simulink model "ctrl_typeB"  (R2016b)
settings: Solver=ode45  StartTime=0.0  StopTime=10.0  RelTol=1e-3  EnableMultiTasking=on
undefined symbols (not defined in the file): gain_act_GASBF, gain_act_GASF0, gain_act_GASF1, gain_act_LIM, gain_act_LIP, gain_act_LTM, gain_act_PIM, gain_act_PTM, gain_act_RIM, gain_act_TIM, gain_act_TIP, gain_act_VIM, gain_act_YIM, gain_act_YIP, gain_act_YTM, gain_GASBF, gain_GASF0, gain_GASF1, gain_global_LIM, gain_global_LIP, gain_global_LTM, gain_LIM, gain_LIP, gain_LTM, gain_oplev_PIM, gain_oplev_YIM, gain_PIM, gain_PTM, gain_RIM, gain_TIM, gain_TIP, gain_VIM, gain_YIM, gain_YIP, gain_YTM, sys1
libraries: cstblocks x26, simulink x3
settings Model: Creator=TAMA Project  LastModifiedBy=miyo
settings DataIOCC: LimitDataPoints=on  SaveFormat=Array  SignalLoggingSaveFormat=ModelDataLogs
settings OptimizationCC: ExpressionDepthLimit=2147483647  LifeSpan=inf
settings DebuggingCC: UnderspecifiedInitializationDetection=Classic  MergeDetectMultiDrivingBlocksExec=none  FcnCallInpInsideContextMsg=warning  StateNameClashWarn=warning  SFUnexpectedBacktrackingDiag=warning  SFNoUnconditionalDefaultTransitionDiag=warning  SFExecutionAtInitializationDiag=none
settings HardwareCC: ProdBitPerPointer=32  ProdBitPerSizeT=32  ProdBitPerPtrDiffT=32  ProdLargestAtomicFloat=None  ProdIntDivRoundTo=Undefined  ProdEndianess=Unspecified  ProdWordSize=32  ProdHWDeviceType=32-bit Generic
settings ModelReferenceCC: PropagateSignalLabelsOutOfModel=off
settings GRTTargetCC: TargetLangStandard=C89/C90 (ANSI)  GeneratePreprocessorConditionals=Disable all  CombineOutputUpdateFcns=off  GRTInterface=on
settings ConfigComp: CovMetricSettings=dw  CovHtmlReporting=on  CovSaveCumulativeToWorkspaceVar=on  CovSaveSingleToWorkspaceVar=on  CovExternalEMLEnable=off  CovSFcnEnable=off

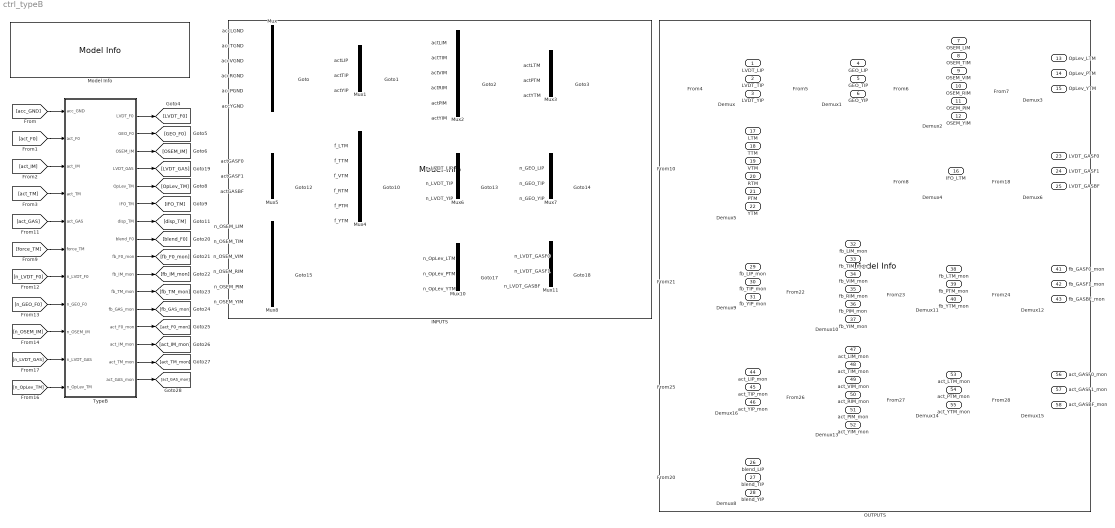
== system ctrl_typeB ==
  accLGND : Inport
  accTGND : Inport  Port=2
  accVGND : Inport  Port=3
  accRGND : Inport  Port=4
  accPGND : Inport  Port=5
  accYGND : Inport  Port=6
  actLIP : Inport  Port=7
  actTIP : Inport  Port=8
  actYIP : Inport  Port=9
  actLIM : Inport  Port=10
  actTIM : Inport  Port=11
  actVIM : Inport  Port=12
  actRIM : Inport  Port=13
  actPIM : Inport  Port=14
  actYIM : Inport  Port=15
  actLTM : Inport  Port=16
  actPTM : Inport  Port=17
  actYTM : Inport  Port=18
  f_LTM : Inport  Port=19
  f_TTM : Inport  Port=20
  f_VTM : Inport  Port=21
  f_RTM : Inport  Port=22
  f_PTM : Inport  Port=23
  f_YTM : Inport  Port=24
  actGASF0 : Inport  Port=25
  actGASF1 : Inport  Port=26
  actGASBF : Inport  Port=27
  n_LVDT_LIP : Inport  Port=28
  n_LVDT_TIP : Inport  Port=29
  n_LVDT_YIP : Inport  Port=30
  n_GEO_LIP : Inport  Port=31
  n_GEO_TIP : Inport  Port=32
  n_GEO_YIP : Inport  Port=33
  n_OSEM_LIM : Inport  Port=34
  n_OSEM_TIM : Inport  Port=35
  n_OSEM_VIM : Inport  Port=36
  n_OSEM_RIM : Inport  Port=37
  n_OSEM_PIM : Inport  Port=38
  n_OSEM_YIM : Inport  Port=39
  n_OpLev_LTM : Inport  Port=40
  n_OpLev_PTM : Inport  Port=41
  n_OpLev_YTM : Inport  Port=42
  n_LVDT_GASF0 : Inport  Port=43
  n_LVDT_GASF1 : Inport  Port=44
  n_LVDT_GASBF : Inport  Port=45
  Demux{,1,3,6,8..9,11..12,14..16} (11 alike) : Demux  Outputs=3
  Demux{2,5,10,13} (4 alike) : Demux  Outputs=6
  Demux4 : Demux  Outputs=1
  INPUTS : simulink/Model-Wide Utilities/Model Info  Frame=on  DisplayStringWithTags=Model Info  HorizontalTextAlignment=Left  LeftAlignmentValue=0.02  SourceBlockDiagram=ctrl_typeB  TagMaxNumber=20
  Model Info : simulink/Model-Wide Utilities/Model Info  Frame=on  DisplayStringWithTags=|  HorizontalTextAlignment=Left  LeftAlignmentValue=0.02  SourceBlockDiagram=ctrl_typeB  TagMaxNumber=20
      | [MODEL INFORMATION]
      | 
      | ModelName: %<ModelName>
      | LastUpdate : %<LastModificationDate>
      | 
      | TypeB1 prototype control model
  Mux{,2,4,8} (4 alike) : Mux  Inputs=6
  Mux{1,3,5..7,10..11} (7 alike) : Mux  Inputs=3
  OUTPUTS : simulink/Model-Wide Utilities/Model Info  Frame=on  DisplayStringWithTags=Model Info  HorizontalTextAlignment=Left  LeftAlignmentValue=0.02  SourceBlockDiagram=ctrl_typeB  TagMaxNumber=20
  TypeB : Subsystem
  LVDT_LIP : Outport
  LVDT_TIP : Outport  Port=2
  LVDT_YIP : Outport  Port=3
  GEO_LIP : Outport  Port=4
  GEO_TIP : Outport  Port=5
  GEO_YIP : Outport  Port=6
  OSEM_LIM : Outport  Port=7
  OSEM_TIM : Outport  Port=8
  OSEM_VIM : Outport  Port=9
  OSEM_RIM : Outport  Port=10
  OSEM_PIM : Outport  Port=11
  OSEM_YIM : Outport  Port=12
  OpLev_LTM : Outport  Port=13
  OpLev_PTM : Outport  Port=14
  OpLev_YTM : Outport  Port=15
  IFO_LTM : Outport  Port=16
  LTM : Outport  Port=17
  TTM : Outport  Port=18
  VTM : Outport  Port=19
  RTM : Outport  Port=20
  PTM : Outport  Port=21
  YTM : Outport  Port=22
  LVDT_GASF0 : Outport  Port=23
  LVDT_GASF1 : Outport  Port=24
  LVDT_GASBF : Outport  Port=25
  blend_LIP : Outport  Port=26
  blend_TIP : Outport  Port=27
  blend_YIP : Outport  Port=28
  fb_LIP_mon : Outport  Port=29
  fb_TIP_mon : Outport  Port=30
  fb_YIP_mon : Outport  Port=31
  fb_LIM_mon : Outport  Port=32
  fb_TIM_mon : Outport  Port=33
  fb_VIM_mon : Outport  Port=34
  fb_RIM_mon : Outport  Port=35
  fb_PIM_mon : Outport  Port=36
  fb_YIM_mon : Outport  Port=37
  fb_LTM_mon : Outport  Port=38
  fb_PTM_mon : Outport  Port=39
  fb_YTM_mon : Outport  Port=40
  fb_GASF0_mon : Outport  Port=41
  fb_GASF1_mon : Outport  Port=42
  fb_GASBF_mon : Outport  Port=43
  act_LIP_mon : Outport  Port=44
  act_TIP_mon : Outport  Port=45
  act_YIP_mon : Outport  Port=46
  act_LIM_mon : Outport  Port=47
  act_TIM_mon : Outport  Port=48
  act_VIM_mon : Outport  Port=49
  act_RIM_mon : Outport  Port=50
  act_PIM_mon : Outport  Port=51
  act_YIM_mon : Outport  Port=52
  act_LTM_mon : Outport  Port=53
  act_PTM_mon : Outport  Port=54
  act_YTM_mon : Outport  Port=55
  act_GASF0_mon : Outport  Port=56
  act_GASF1_mon : Outport  Port=57
  act_GASBF_mon : Outport  Port=58
  wires:
  accLGND/1 -> Mux/1
  accTGND/1 -> Mux/2
  accVGND/1 -> Mux/3
  accRGND/1 -> Mux/4
  accPGND/1 -> Mux/5
  accYGND/1 -> Mux/6
  Mux/1 -> [acc_GND]
  actLIP/1 -> Mux1/1
  actTIP/1 -> Mux1/2
  actYIP/1 -> Mux1/3
  Mux1/1 -> [act_F0]
  actLIM/1 -> Mux2/1
  actTIM/1 -> Mux2/2
  actVIM/1 -> Mux2/3
  actRIM/1 -> Mux2/4
  actPIM/1 -> Mux2/5
  actYIM/1 -> Mux2/6
  Mux2/1 -> [act_IM]
  actLTM/1 -> Mux3/1
  actPTM/1 -> Mux3/2
  actYTM/1 -> Mux3/3
  Mux3/1 -> [act_TM]
  [acc_GND] -> TypeB/1(acc_GND)
  [act_F0] -> TypeB/2(act_F0)
  [act_IM] -> TypeB/3(act_IM)
  [act_TM] -> TypeB/4(act_TM)
  TypeB/1(LVDT_F0) -> [LVDT_F0]
  TypeB/2(GEO_F0) -> [GEO_F0]
  TypeB/3(OSEM_IM) -> [OSEM_IM]
  TypeB/5(OpLev_TM) -> [OpLev_TM]
  [LVDT_F0] -> Demux/1
  Demux/1 -> LVDT_LIP/1
  Demux/2 -> LVDT_TIP/1
  Demux/3 -> LVDT_YIP/1
  [GEO_F0] -> Demux1/1
  Demux1/1 -> GEO_LIP/1
  Demux1/2 -> GEO_TIP/1
  Demux1/3 -> GEO_YIP/1
  [OSEM_IM] -> Demux2/1
  Demux2/1 -> OSEM_LIM/1
  Demux2/2 -> OSEM_TIM/1
  Demux2/3 -> OSEM_VIM/1
  Demux2/4 -> OSEM_RIM/1
  Demux2/5 -> OSEM_PIM/1
  Demux2/6 -> OSEM_YIM/1
  [OpLev_TM] -> Demux3/1
  TypeB/6(IFO_TM) -> [IFO_TM]
  [IFO_TM] -> Demux4/1
  Demux4/1 -> IFO_LTM/1
  f_LTM/1 -> Mux4/1
  f_TTM/1 -> Mux4/2
  f_VTM/1 -> Mux4/3
  Mux4/1 -> [force_TM]
  f_YTM/1 -> Mux4/6
  f_PTM/1 -> Mux4/5
  f_RTM/1 -> Mux4/4
  [force_TM] -> TypeB/6(force_TM)
  TypeB/7(disp_TM) -> [disp_TM]
  [disp_TM] -> Demux5/1
  Demux5/1 -> LTM/1
  Demux5/2 -> TTM/1
  Demux5/3 -> VTM/1
  Demux5/4 -> RTM/1
  Demux5/5 -> PTM/1
  Demux5/6 -> YTM/1
  actGASF0/1 -> Mux5/1
  actGASF1/1 -> Mux5/2
  actGASBF/1 -> Mux5/3
  Mux5/1 -> [act_GAS]
  [act_GAS] -> TypeB/5(act_GAS)
  n_LVDT_LIP/1 -> Mux6/1
  n_LVDT_TIP/1 -> Mux6/2
  n_LVDT_YIP/1 -> Mux6/3
  Mux6/1 -> [n_LVDT_F0]
  n_GEO_LIP/1 -> Mux7/1
  n_GEO_TIP/1 -> Mux7/2
  n_GEO_YIP/1 -> Mux7/3
  Mux7/1 -> [n_GEO_F0]
  n_OSEM_LIM/1 -> Mux8/1
  n_OSEM_TIM/1 -> Mux8/2
  n_OSEM_VIM/1 -> Mux8/3
  n_OSEM_RIM/1 -> Mux8/4
  n_OSEM_PIM/1 -> Mux8/5
  n_OSEM_YIM/1 -> Mux8/6
  Mux8/1 -> [n_OSEM_IM]
  Mux10/1 -> [n_OpLev_TM]
  [n_LVDT_F0] -> TypeB/7(n_LVDT_F0)
  [n_GEO_F0] -> TypeB/8(n_GEO_F0)
  [n_OSEM_IM] -> TypeB/9(n_OSEM_IM)
  n_LVDT_GASF0/1 -> Mux11/1
  n_LVDT_GASF1/1 -> Mux11/2
  n_LVDT_GASBF/1 -> Mux11/3
  Mux11/1 -> [n_LVDT_GAS]
  [n_LVDT_GAS] -> TypeB/10(n_LVDT_GAS)
  TypeB/4(LVDT_GAS) -> [LVDT_GAS]
  [LVDT_GAS] -> Demux6/1
  Demux6/1 -> LVDT_GASF0/1
  Demux6/2 -> LVDT_GASF1/1
  Demux6/3 -> LVDT_GASBF/1
  [n_OpLev_TM] -> TypeB/11(n_OpLev_TM)
  TypeB/8(blend_F0) -> [blend_F0]
  TypeB/9(fb_F0_mon) -> [fb_F0_mon]
  TypeB/10(fb_IM_mon) -> [fb_IM_mon]
  TypeB/11(fb_TM_mon) -> [fb_TM_mon]
  TypeB/12(fb_GAS_mon) -> [fb_GAS_mon]
  TypeB/13(act_F0_mon) -> [act_F0_mon]
  TypeB/14(act_IM_mon) -> [act_IM_mon]
  TypeB/15(act_TM_mon) -> [act_TM_mon]
  TypeB/16(act_GAS_mon) -> [act_GAS_mon]
  [blend_F0] -> Demux8/1
  Demux8/1 -> blend_LIP/1
  Demux8/2 -> blend_TIP/1
  Demux8/3 -> blend_YIP/1
  [fb_F0_mon] -> Demux9/1
  Demux9/1 -> fb_LIP_mon/1
  Demux9/2 -> fb_TIP_mon/1
  Demux9/3 -> fb_YIP_mon/1
  [fb_IM_mon] -> Demux10/1
  Demux10/1 -> fb_LIM_mon/1
  Demux10/2 -> fb_TIM_mon/1
  Demux10/3 -> fb_VIM_mon/1
  Demux10/4 -> fb_RIM_mon/1
  Demux10/5 -> fb_PIM_mon/1
  Demux10/6 -> fb_YIM_mon/1
  [fb_TM_mon] -> Demux11/1
  Demux11/1 -> fb_LTM_mon/1
  Demux11/2 -> fb_PTM_mon/1
  Demux11/3 -> fb_YTM_mon/1
  [fb_GAS_mon] -> Demux12/1
  Demux12/1 -> fb_GASF0_mon/1
  Demux12/2 -> fb_GASF1_mon/1
  Demux12/3 -> fb_GASBF_mon/1
  [act_F0_mon] -> Demux16/1
  Demux16/1 -> act_LIP_mon/1
  Demux16/2 -> act_TIP_mon/1
  Demux16/3 -> act_YIP_mon/1
  [act_IM_mon] -> Demux13/1
  Demux13/1 -> act_LIM_mon/1
  Demux13/2 -> act_TIM_mon/1
  Demux13/3 -> act_VIM_mon/1
  Demux13/4 -> act_RIM_mon/1
  Demux13/5 -> act_PIM_mon/1
  Demux13/6 -> act_YIM_mon/1
  [act_TM_mon] -> Demux14/1
  Demux14/1 -> act_LTM_mon/1
  Demux14/2 -> act_PTM_mon/1
  Demux14/3 -> act_YTM_mon/1
  [act_GAS_mon] -> Demux15/1
  Demux15/1 -> act_GASF0_mon/1
  Demux15/2 -> act_GASF1_mon/1
  Demux15/3 -> act_GASBF_mon/1
  n_OpLev_LTM/1 -> Mux10/1
  n_OpLev_PTM/1 -> Mux10/2
  n_OpLev_YTM/1 -> Mux10/3
  Demux3/1 -> OpLev_LTM/1
  Demux3/2 -> OpLev_PTM/1
  Demux3/3 -> OpLev_YTM/1

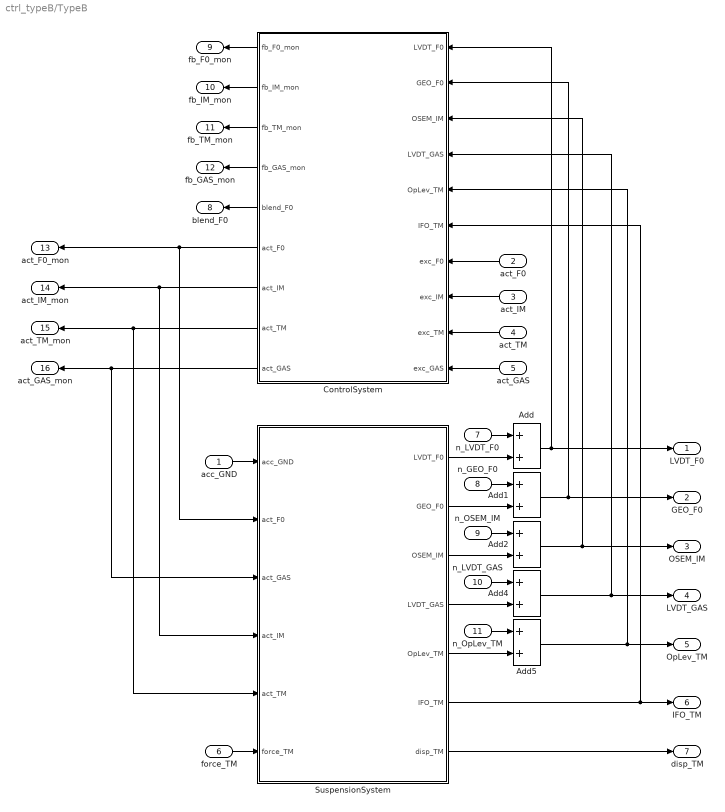
== system ctrl_typeB/TypeB ==
  acc_GND : Inport
  act_F0 : Inport  Port=2
  act_IM : Inport  Port=3
  act_TM : Inport  Port=4
  act_GAS : Inport  Port=5
  force_TM : Inport  Port=6
  n_LVDT_F0 : Inport  Port=7
  n_GEO_F0 : Inport  Port=8
  n_OSEM_IM : Inport  Port=9
  n_LVDT_GAS : Inport  Port=10
  n_OpLev_TM : Inport  Port=11
  Add{,1..2,4..5} (5 alike) : Sum
  ControlSystem : Subsystem
  SuspensionSystem : Subsystem
  LVDT_F0 : Outport
  GEO_F0 : Outport  Port=2
  OSEM_IM : Outport  Port=3
  LVDT_GAS : Outport  Port=4
  OpLev_TM : Outport  Port=5
  IFO_TM : Outport  Port=6
  disp_TM : Outport  Port=7
  blend_F0 : Outport  Port=8
  fb_F0_mon : Outport  Port=9
  fb_IM_mon : Outport  Port=10
  fb_TM_mon : Outport  Port=11
  fb_GAS_mon : Outport  Port=12
  act_F0_mon : Outport  Port=13
  act_IM_mon : Outport  Port=14
  act_TM_mon : Outport  Port=15
  act_GAS_mon : Outport  Port=16
  wires:
  acc_GND/1 -> SuspensionSystem/1(acc_GND)
  force_TM/1 -> SuspensionSystem/6(force_TM)
  SuspensionSystem/7(disp_TM) -> disp_TM/1
  SuspensionSystem/1(LVDT_F0) -> Add/2
  SuspensionSystem/2(GEO_F0) -> Add1/2
  n_GEO_F0/1 -> Add1/1
  n_LVDT_F0/1 -> Add/1
  SuspensionSystem/3(OSEM_IM) -> Add2/2
  n_OSEM_IM/1 -> Add2/1
  SuspensionSystem/6(IFO_TM) -> IFO_TM/1, ControlSystem/6(IFO_TM)
  Add/1 -> LVDT_F0/1, ControlSystem/1(LVDT_F0)
  Add1/1 -> ControlSystem/2(GEO_F0), GEO_F0/1
  Add2/1 -> ControlSystem/3(OSEM_IM), OSEM_IM/1
  n_LVDT_GAS/1 -> Add4/1
  SuspensionSystem/4(LVDT_GAS) -> Add4/2
  n_OpLev_TM/1 -> Add5/1
  SuspensionSystem/5(OpLev_TM) -> Add5/2
  Add4/1 -> ControlSystem/4(LVDT_GAS), LVDT_GAS/1
  Add5/1 -> ControlSystem/5(OpLev_TM), OpLev_TM/1
  ControlSystem/5(blend_F0) -> blend_F0/1
  act_GAS/1 -> ControlSystem/10(exc_GAS)
  act_TM/1 -> ControlSystem/9(exc_TM)
  act_IM/1 -> ControlSystem/8(exc_IM)
  act_F0/1 -> ControlSystem/7(exc_F0)
  ControlSystem/6(act_F0) -> act_F0_mon/1, SuspensionSystem/2(act_F0)
  ControlSystem/7(act_IM) -> SuspensionSystem/4(act_IM), act_IM_mon/1
  ControlSystem/8(act_TM) -> act_TM_mon/1, SuspensionSystem/5(act_TM)
  ControlSystem/9(act_GAS) -> SuspensionSystem/3(act_GAS), act_GAS_mon/1
  ControlSystem/1(fb_F0_mon) -> fb_F0_mon/1
  ControlSystem/2(fb_IM_mon) -> fb_IM_mon/1
  ControlSystem/3(fb_TM_mon) -> fb_TM_mon/1
  ControlSystem/4(fb_GAS_mon) -> fb_GAS_mon/1

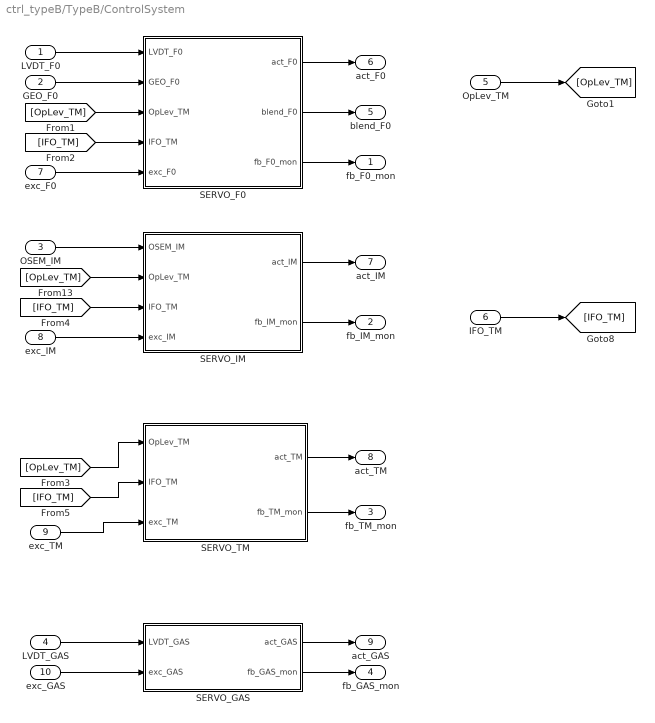
== system ctrl_typeB/TypeB/ControlSystem ==
  LVDT_F0 : Inport
  GEO_F0 : Inport  Port=2
  OSEM_IM : Inport  Port=3
  LVDT_GAS : Inport  Port=4
  OpLev_TM : Inport  Port=5
  IFO_TM : Inport  Port=6
  exc_F0 : Inport  Port=7
  exc_IM : Inport  Port=8
  exc_TM : Inport  Port=9
  exc_GAS : Inport  Port=10
  SERVO_F0 : Subsystem
  SERVO_GAS : Subsystem
  SERVO_IM : Subsystem
  SERVO_TM : Subsystem
  fb_F0_mon : Outport
  fb_IM_mon : Outport  Port=2
  fb_TM_mon : Outport  Port=3
  fb_GAS_mon : Outport  Port=4
  blend_F0 : Outport  Port=5
  act_F0 : Outport  Port=6
  act_IM : Outport  Port=7
  act_TM : Outport  Port=8
  act_GAS : Outport  Port=9
  wires:
  IFO_TM/1 -> [IFO_TM]
  LVDT_F0/1 -> SERVO_F0/1(LVDT_F0)
  GEO_F0/1 -> SERVO_F0/2(GEO_F0)
  SERVO_F0/1(act_F0) -> act_F0/1
  SERVO_IM/1(act_IM) -> act_IM/1
  OSEM_IM/1 -> SERVO_IM/1(OSEM_IM)
  LVDT_GAS/1 -> SERVO_GAS/1(LVDT_GAS)
  SERVO_GAS/1(act_GAS) -> act_GAS/1
  SERVO_TM/1(act_TM) -> act_TM/1
  OpLev_TM/1 -> [OpLev_TM]
  [OpLev_TM] -> SERVO_IM/2(OpLev_TM)
  [IFO_TM] -> SERVO_F0/4(IFO_TM)
  [IFO_TM] -> SERVO_IM/3(IFO_TM)
  [OpLev_TM] -> SERVO_F0/3(OpLev_TM)
  SERVO_F0/2(blend_F0) -> blend_F0/1
  exc_F0/1 -> SERVO_F0/5(exc_F0)
  exc_IM/1 -> SERVO_IM/4(exc_IM)
  exc_GAS/1 -> SERVO_GAS/2(exc_GAS)
  SERVO_F0/3(fb_F0_mon) -> fb_F0_mon/1
  SERVO_IM/2(fb_IM_mon) -> fb_IM_mon/1
  SERVO_TM/2(fb_TM_mon) -> fb_TM_mon/1
  SERVO_GAS/2(fb_GAS_mon) -> fb_GAS_mon/1
  [OpLev_TM] -> SERVO_TM/1(OpLev_TM)
  [IFO_TM] -> SERVO_TM/2(IFO_TM)
  exc_TM/1 -> SERVO_TM/3(exc_TM)

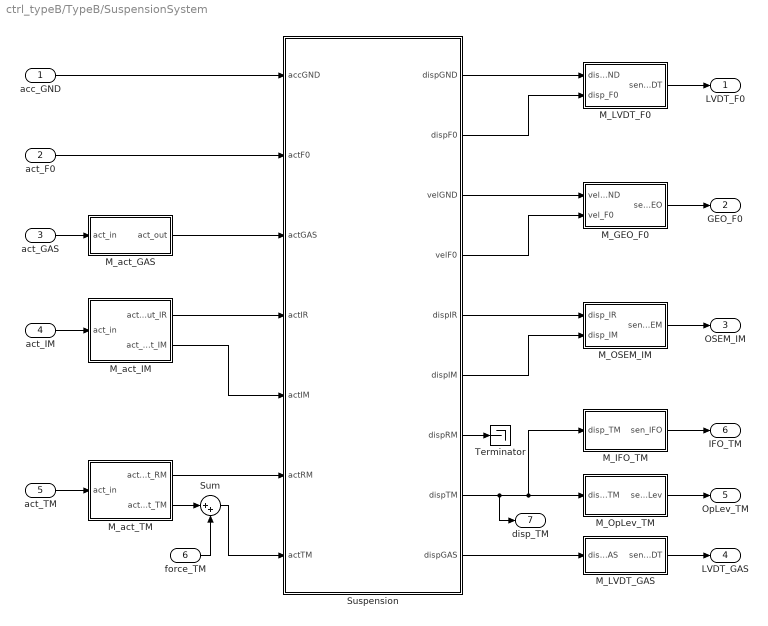
== system ctrl_typeB/TypeB/SuspensionSystem ==
  acc_GND : Inport
  act_F0 : Inport  Port=2
  act_GAS : Inport  Port=3
  act_IM : Inport  Port=4
  act_TM : Inport  Port=5
  force_TM : Inport  Port=6
  M_GEO_F0 : Subsystem
  M_IFO_TM : Subsystem
  M_LVDT_F0 : Subsystem
  M_LVDT_GAS : Subsystem
  M_OSEM_IM : Subsystem
  M_OpLev_TM : Subsystem
  M_act_GAS : Subsystem
  M_act_IM : Subsystem
  M_act_TM : Subsystem
  Sum : Sum  Inputs=|++
  Suspension : Subsystem
  Terminator : Terminator
  LVDT_F0 : Outport
  GEO_F0 : Outport  Port=2
  OSEM_IM : Outport  Port=3
  LVDT_GAS : Outport  Port=4
  OpLev_TM : Outport  Port=5
  IFO_TM : Outport  Port=6
  disp_TM : Outport  Port=7
  wires:
  acc_GND/1 -> Suspension/1(accGND)
  act_F0/1 -> Suspension/2(actF0)
  act_IM/1 -> M_act_IM/1(act_in)
  M_act_IM/1(act_out_IR) -> Suspension/4(actIR)
  M_act_IM/2(act_out_IM) -> Suspension/5(actIM)
  act_TM/1 -> M_act_TM/1(act_in)
  Sum/1 -> Suspension/7(actTM)
  M_act_TM/2(act_out_TM) -> Sum/1
  force_TM/1 -> Sum/2
  M_act_GAS/1(act_out) -> Suspension/3(actGAS)
  act_GAS/1 -> M_act_GAS/1(act_in)
  Suspension/1(dispGND) -> M_LVDT_F0/1(disp_GND)
  Suspension/2(dispF0) -> M_LVDT_F0/2(disp_F0)
  M_LVDT_F0/1(sen_LVDT) -> LVDT_F0/1
  Suspension/3(velGND) -> M_GEO_F0/1(vel_GND)
  Suspension/4(velF0) -> M_GEO_F0/2(vel_F0)
  M_GEO_F0/1(sen_GEO) -> GEO_F0/1
  Suspension/5(dispIR) -> M_OSEM_IM/1(disp_IR)
  Suspension/6(dispIM) -> M_OSEM_IM/2(disp_IM)
  M_OSEM_IM/1(sen_OSEM) -> OSEM_IM/1
  Suspension/8(dispTM) -> disp_TM/1, M_IFO_TM/1(disp_TM), M_OpLev_TM/1(disp_TM)
  Suspension/9(dispGAS) -> M_LVDT_GAS/1(disp_GAS)
  M_LVDT_GAS/1(sen_LVDT) -> LVDT_GAS/1
  M_IFO_TM/1(sen_IFO) -> IFO_TM/1
  M_OpLev_TM/1(sen_OpLev) -> OpLev_TM/1
  Suspension/7(dispRM) -> Terminator/1
  M_act_TM/1(act_out_RM) -> Suspension/6(actRM)

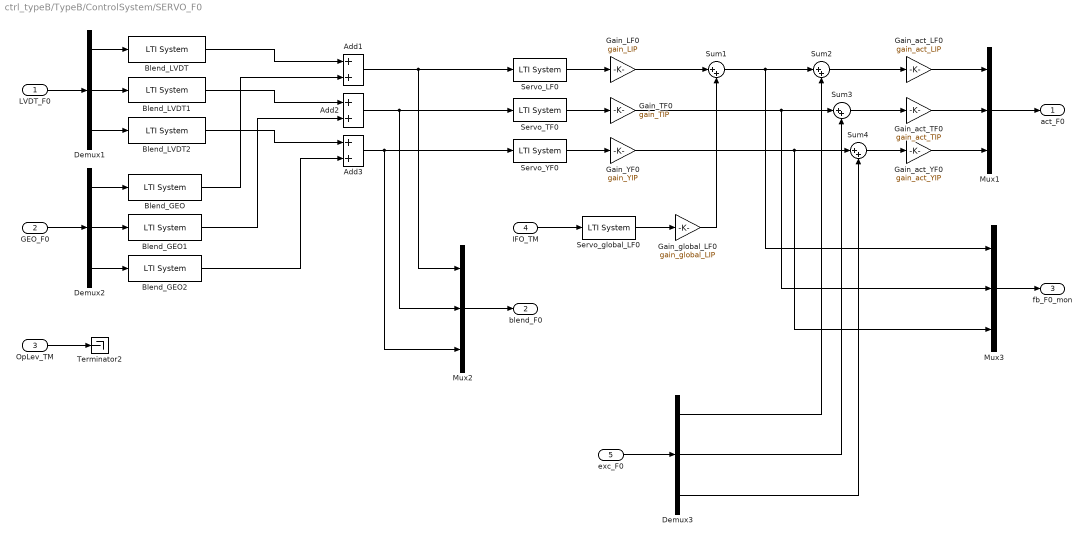
== system ctrl_typeB/TypeB/ControlSystem/SERVO_F0 ==
  LVDT_F0 : Inport
  GEO_F0 : Inport  Port=2
  OpLev_TM : Inport  Port=3
  IFO_TM : Inport  Port=4
  exc_F0 : Inport  Port=5
  Add1 : Sum
  Add2 : Sum
  Add3 : Sum
  Blend_GEO : cstblocks/LTI System  sys=blend_GEO  IC=[]
  Blend_GEO1 : cstblocks/LTI System  sys=blend_GEO  IC=[]
  Blend_GEO2 : cstblocks/LTI System  sys=blend_GEO  IC=[]
  Blend_LVDT : cstblocks/LTI System  sys=blend_LVDT  IC=[]
  Blend_LVDT1 : cstblocks/LTI System  sys=blend_LVDT  IC=[]
  Blend_LVDT2 : cstblocks/LTI System  sys=blend_LVDT  IC=[]
  Demux1 : Demux  Outputs=3
  Demux2 : Demux  Outputs=3
  Demux3 : Demux  Outputs=3
  Gain_LF0 : Gain  Gain=gain_LIP
  Gain_TF0 : Gain  Gain=gain_TIP
  Gain_YF0 : Gain  Gain=gain_YIP
  Gain_act_LF0 : Gain  Gain=gain_act_LIP
  Gain_act_TF0 : Gain  Gain=gain_act_TIP
  Gain_act_YF0 : Gain  Gain=gain_act_YIP
  Gain_global_LF0 : Gain  Gain=gain_global_LIP
  Mux1 : Mux  Inputs=3
  Mux2 : Mux  Inputs=3
  Mux3 : Mux  Inputs=3
  Servo_LF0 : cstblocks/LTI System  sys=servo_LIP  IC=[]
  Servo_TF0 : cstblocks/LTI System  sys=servo_TIP  IC=[]
  Servo_YF0 : cstblocks/LTI System  sys=servo_YIP  IC=[]
  Servo_global_LF0 : cstblocks/LTI System  sys=servo_global_LIP  IC=[]
  Sum{1..4} (4 alike) : Sum  Inputs=|++
  Terminator2 : Terminator
  act_F0 : Outport
  blend_F0 : Outport  Port=2
  fb_F0_mon : Outport  Port=3
  wires:
  Blend_LVDT/1 -> Add1/1
  IFO_TM/1 -> Servo_global_LF0/1
  Mux1/1 -> act_F0/1
  LVDT_F0/1 -> Demux1/1
  GEO_F0/1 -> Demux2/1
  Demux1/1 -> Blend_LVDT/1
  Demux1/2 -> Blend_LVDT1/1
  Demux1/3 -> Blend_LVDT2/1
  Demux2/1 -> Blend_GEO/1
  Demux2/2 -> Blend_GEO1/1
  Demux2/3 -> Blend_GEO2/1
  Blend_LVDT1/1 -> Add2/1
  Blend_LVDT2/1 -> Add3/1
  Blend_GEO/1 -> Add1/2
  Blend_GEO1/1 -> Add2/2
  Blend_GEO2/1 -> Add3/2
  Add1/1 -> Servo_LF0/1, Mux2/1
  Add2/1 -> Servo_TF0/1, Mux2/2
  Add3/1 -> Servo_YF0/1, Mux2/3
  OpLev_TM/1 -> Terminator2/1
  Servo_LF0/1 -> Gain_LF0/1
  Gain_LF0/1 -> Sum1/1
  Servo_TF0/1 -> Gain_TF0/1
  Servo_YF0/1 -> Gain_YF0/1
  Servo_global_LF0/1 -> Gain_global_LF0/1
  Gain_global_LF0/1 -> Sum1/2
  Gain_act_LF0/1 -> Mux1/1
  Gain_act_TF0/1 -> Mux1/2
  Gain_act_YF0/1 -> Mux1/3
  Mux2/1 -> blend_F0/1
  Gain_TF0/1 -> Mux3/2, Sum3/1
  Sum2/1 -> Gain_act_LF0/1
  Sum1/1 -> Mux3/1, Sum2/1
  Sum3/1 -> Gain_act_TF0/1
  exc_F0/1 -> Demux3/1
  Demux3/1 -> Sum2/2
  Demux3/2 -> Sum3/2
  Demux3/3 -> Sum4/2
  Gain_YF0/1 -> Mux3/3, Sum4/1
  Sum4/1 -> Gain_act_YF0/1
  Mux3/1 -> fb_F0_mon/1

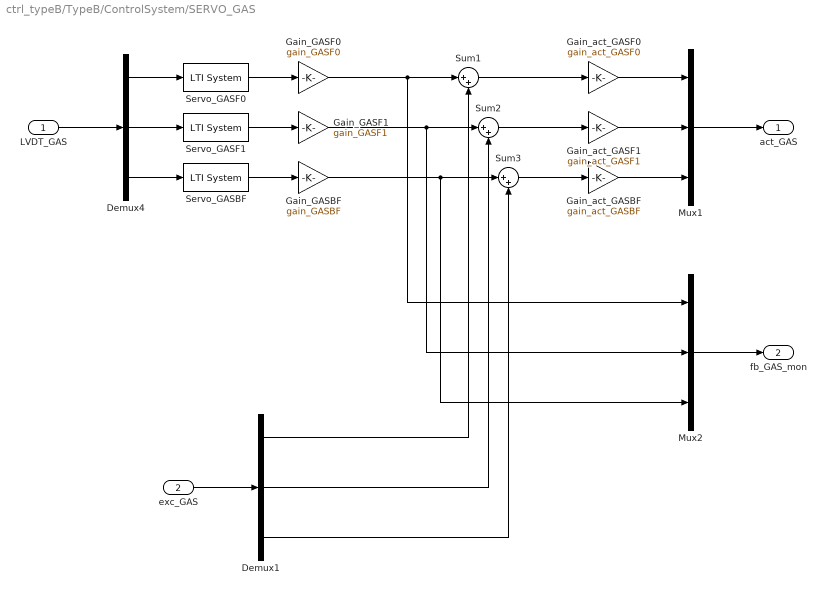
== system ctrl_typeB/TypeB/ControlSystem/SERVO_GAS ==
  LVDT_GAS : Inport
  exc_GAS : Inport  Port=2
  Demux1 : Demux  Outputs=3
  Demux4 : Demux  Outputs=3
  Gain_GASBF : Gain  Gain=gain_GASBF
  Gain_GASF0 : Gain  Gain=gain_GASF0
  Gain_GASF1 : Gain  Gain=gain_GASF1
  Gain_act_GASBF : Gain  Gain=gain_act_GASBF
  Gain_act_GASF0 : Gain  Gain=gain_act_GASF0
  Gain_act_GASF1 : Gain  Gain=gain_act_GASF1
  Mux1 : Mux  Inputs=3
  Mux2 : Mux  Inputs=3
  Servo_GASBF : cstblocks/LTI System  sys=servo_GASBF  IC=[]
  Servo_GASF0 : cstblocks/LTI System  sys=servo_GASF0  IC=[]
  Servo_GASF1 : cstblocks/LTI System  sys=servo_GASF1  IC=[]
  Sum1 : Sum  Inputs=|++
  Sum2 : Sum  Inputs=|++
  Sum3 : Sum  Inputs=|++
  act_GAS : Outport
  fb_GAS_mon : Outport  Port=2
  wires:
  Demux4/1 -> Servo_GASF0/1
  Demux4/2 -> Servo_GASF1/1
  Demux4/3 -> Servo_GASBF/1
  Servo_GASF0/1 -> Gain_GASF0/1
  Servo_GASF1/1 -> Gain_GASF1/1
  Servo_GASBF/1 -> Gain_GASBF/1
  Gain_act_GASF0/1 -> Mux1/1
  Gain_act_GASF1/1 -> Mux1/2
  Gain_act_GASBF/1 -> Mux1/3
  LVDT_GAS/1 -> Demux4/1
  Mux1/1 -> act_GAS/1
  exc_GAS/1 -> Demux1/1
  Gain_GASF0/1 -> Mux2/1, Sum1/1
  Sum1/1 -> Gain_act_GASF0/1
  Gain_GASF1/1 -> Mux2/2, Sum2/1
  Sum2/1 -> Gain_act_GASF1/1
  Gain_GASBF/1 -> Mux2/3, Sum3/1
  Sum3/1 -> Gain_act_GASBF/1
  Demux1/1 -> Sum1/2
  Demux1/2 -> Sum2/2
  Demux1/3 -> Sum3/2
  Mux2/1 -> fb_GAS_mon/1

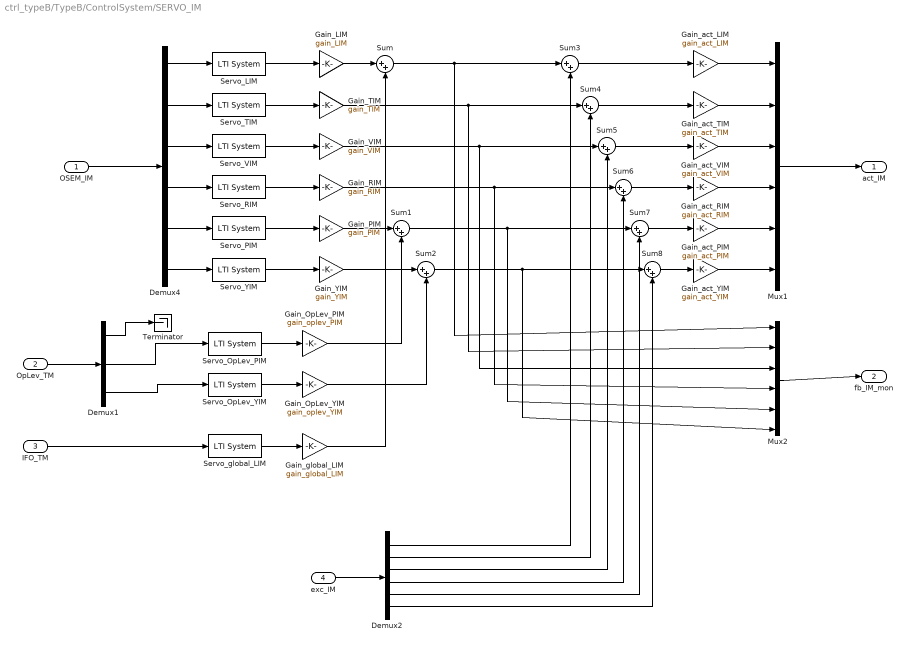
== system ctrl_typeB/TypeB/ControlSystem/SERVO_IM ==
  OSEM_IM : Inport
  OpLev_TM : Inport  Port=2
  IFO_TM : Inport  Port=3
  exc_IM : Inport  Port=4
  Demux1 : Demux  Outputs=3
  Demux2 : Demux  Outputs=6
  Demux4 : Demux  Outputs=6
  Gain_LIM : Gain  Gain=gain_LIM
  Gain_OpLev_PIM : Gain  Gain=gain_oplev_PIM
  Gain_OpLev_YIM : Gain  Gain=gain_oplev_YIM
  Gain_PIM : Gain  Gain=gain_PIM
  Gain_RIM : Gain  Gain=gain_RIM
  Gain_TIM : Gain  Gain=gain_TIM
  Gain_VIM : Gain  Gain=gain_VIM
  Gain_YIM : Gain  Gain=gain_YIM
  Gain_act_LIM : Gain  Gain=gain_act_LIM
  Gain_act_PIM : Gain  Gain=gain_act_PIM
  Gain_act_RIM : Gain  Gain=gain_act_RIM
  Gain_act_TIM : Gain  Gain=gain_act_TIM
  Gain_act_VIM : Gain  Gain=gain_act_VIM
  Gain_act_YIM : Gain  Gain=gain_act_YIM
  Gain_global_LIM : Gain  Gain=gain_global_LIM
  Mux1 : Mux  Inputs=6
  Mux2 : Mux  Inputs=6
  Servo_LIM : cstblocks/LTI System  sys=servo_LIM  IC=[]
  Servo_OpLev_PIM : cstblocks/LTI System  sys=servo_oplev_PIM  IC=[]
  Servo_OpLev_YIM : cstblocks/LTI System  sys=servo_oplev_YIM  IC=[]
  Servo_PIM : cstblocks/LTI System  sys=servo_PIM  IC=[]
  Servo_RIM : cstblocks/LTI System  sys=servo_RIM  IC=[]
  Servo_TIM : cstblocks/LTI System  sys=servo_TIM  IC=[]
  Servo_VIM : cstblocks/LTI System  sys=servo_VIM  IC=[]
  Servo_YIM : cstblocks/LTI System  sys=servo_YIM  IC=[]
  Servo_global_LIM : cstblocks/LTI System  sys=servo_global_LIM  IC=[]
  Sum{,1..8} (9 alike) : Sum  Inputs=|++
  Terminator : Terminator
  act_IM : Outport
  fb_IM_mon : Outport  Port=2
  wires:
  Demux4/1 -> Servo_LIM/1
  Demux4/2 -> Servo_TIM/1
  Demux4/3 -> Servo_VIM/1
  Servo_LIM/1 -> Gain_LIM/1
  Servo_TIM/1 -> Gain_TIM/1
  Servo_VIM/1 -> Gain_VIM/1
  Mux1/1 -> act_IM/1
  Gain_act_LIM/1 -> Mux1/1
  Gain_act_TIM/1 -> Mux1/2
  Gain_act_VIM/1 -> Mux1/3
  OSEM_IM/1 -> Demux4/1
  Servo_RIM/1 -> Gain_RIM/1
  Servo_PIM/1 -> Gain_PIM/1
  Servo_YIM/1 -> Gain_YIM/1
  Demux4/4 -> Servo_RIM/1
  Demux4/5 -> Servo_PIM/1
  Demux4/6 -> Servo_YIM/1
  Gain_act_RIM/1 -> Mux1/4
  Gain_act_PIM/1 -> Mux1/5
  Gain_act_YIM/1 -> Mux1/6
  OpLev_TM/1 -> Demux1/1
  IFO_TM/1 -> Servo_global_LIM/1
  Gain_LIM/1 -> Sum/1
  Servo_global_LIM/1 -> Gain_global_LIM/1
  Gain_PIM/1 -> Sum1/1
  Gain_YIM/1 -> Sum2/1
  Gain_global_LIM/1 -> Sum/2
  Servo_OpLev_PIM/1 -> Gain_OpLev_PIM/1
  Servo_OpLev_YIM/1 -> Gain_OpLev_YIM/1
  Gain_OpLev_PIM/1 -> Sum1/2
  Gain_OpLev_YIM/1 -> Sum2/2
  Sum/1 -> Sum3/1, Mux2/1
  Sum3/1 -> Gain_act_LIM/1
  Gain_TIM/1 -> Mux2/2, Sum4/1
  Sum4/1 -> Gain_act_TIM/1
  Gain_VIM/1 -> Mux2/3, Sum5/1
  Sum5/1 -> Gain_act_VIM/1
  Gain_RIM/1 -> Sum6/1, Mux2/4
  Sum6/1 -> Gain_act_RIM/1
  Sum1/1 -> Sum7/1, Mux2/5
  Sum7/1 -> Gain_act_PIM/1
  Sum2/1 -> Sum8/1, Mux2/6
  Sum8/1 -> Gain_act_YIM/1
  Demux2/1 -> Sum3/2
  Demux2/2 -> Sum4/2
  Demux2/3 -> Sum5/2
  Demux2/4 -> Sum6/2
  Demux2/5 -> Sum7/2
  Demux2/6 -> Sum8/2
  exc_IM/1 -> Demux2/1
  Mux2/1 -> fb_IM_mon/1
  Demux1/3 -> Servo_OpLev_YIM/1
  Demux1/2 -> Servo_OpLev_PIM/1
  Demux1/1 -> Terminator/1

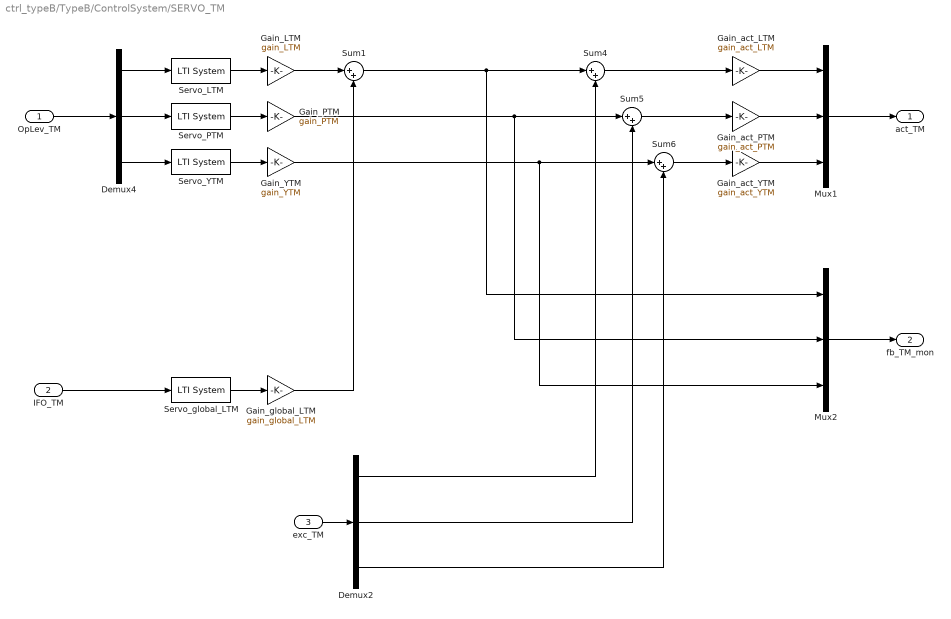
== system ctrl_typeB/TypeB/ControlSystem/SERVO_TM ==
  OpLev_TM : Inport
  IFO_TM : Inport  Port=2
  exc_TM : Inport  Port=3
  Demux2 : Demux  Outputs=3
  Demux4 : Demux  Outputs=3
  Gain_LTM : Gain  Gain=gain_LTM
  Gain_PTM : Gain  Gain=gain_PTM
  Gain_YTM : Gain  Gain=gain_YTM
  Gain_act_LTM : Gain  Gain=gain_act_LTM
  Gain_act_PTM : Gain  Gain=gain_act_PTM
  Gain_act_YTM : Gain  Gain=gain_act_YTM
  Gain_global_LTM : Gain  Gain=gain_global_LTM
  Mux1 : Mux  Inputs=3
  Mux2 : Mux  Inputs=3
  Servo_LTM : cstblocks/LTI System  sys=servo_LTM  IC=[]
  Servo_PTM : cstblocks/LTI System  sys=servo_PTM  IC=[]
  Servo_YTM : cstblocks/LTI System  sys=servo_YTM  IC=[]
  Servo_global_LTM : cstblocks/LTI System  sys=servo_global_LTM  IC=[]
  Sum{1,4..6} (4 alike) : Sum  Inputs=|++
  act_TM : Outport
  fb_TM_mon : Outport  Port=2
  wires:
  Demux4/1 -> Servo_LTM/1
  Demux4/2 -> Servo_PTM/1
  Demux4/3 -> Servo_YTM/1
  Servo_LTM/1 -> Gain_LTM/1
  Servo_PTM/1 -> Gain_PTM/1
  Servo_YTM/1 -> Gain_YTM/1
  OpLev_TM/1 -> Demux4/1
  Mux1/1 -> act_TM/1
  IFO_TM/1 -> Servo_global_LTM/1
  Servo_global_LTM/1 -> Gain_global_LTM/1
  Gain_LTM/1 -> Sum1/1
  Gain_global_LTM/1 -> Sum1/2
  Gain_act_LTM/1 -> Mux1/1
  Gain_act_PTM/1 -> Mux1/2
  Gain_act_YTM/1 -> Mux1/3
  Sum1/1 -> Mux2/1, Sum4/1
  Sum4/1 -> Gain_act_LTM/1
  Gain_PTM/1 -> Mux2/2, Sum5/1
  Sum5/1 -> Gain_act_PTM/1
  Gain_YTM/1 -> Mux2/3, Sum6/1
  Sum6/1 -> Gain_act_YTM/1
  exc_TM/1 -> Demux2/1
  Demux2/1 -> Sum4/2
  Demux2/2 -> Sum5/2
  Demux2/3 -> Sum6/2
  Mux2/1 -> fb_TM_mon/1

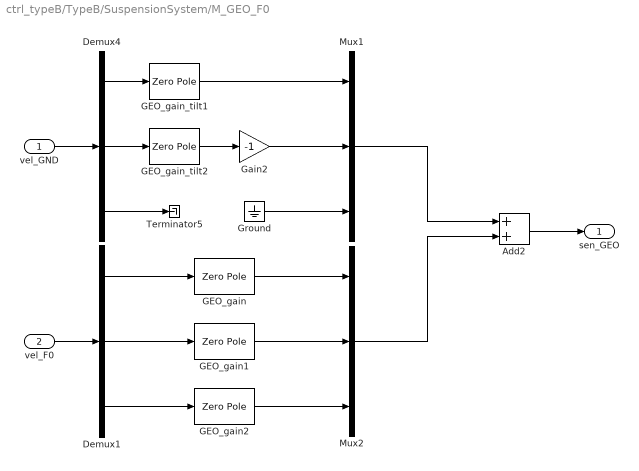
== system ctrl_typeB/TypeB/SuspensionSystem/M_GEO_F0 ==
  vel_GND : Inport
  vel_F0 : Inport  Port=2
  Add2 : Sum
  Demux1 : Demux  Outputs=3
  Demux4 : Demux  Outputs=3
  GEO_gain : ZeroPole  Zeros=[0 0]  Poles=[-2.13+1i*5.19 -2.13-1i*5.19]
  GEO_gain1 : ZeroPole  Zeros=[0 0]  Poles=[-2.13+1i*5.19 -2.13-1i*5.19]
  GEO_gain2 : ZeroPole  Zeros=[0 0]  Poles=[-2.13+1i*5.19 -2.13-1i*5.19]
  GEO_gain_tilt1 : ZeroPole  Zeros=[]  Poles=[-2.13+1i*5.19 -2.13-1i*5.19]
  GEO_gain_tilt2 : ZeroPole  Zeros=[]  Poles=[-2.13+1i*5.19 -2.13-1i*5.19]
  Gain2 : Gain  Gain=-1
  Ground : Ground
  Mux1 : Mux  Inputs=3
  Mux2 : Mux  Inputs=3
  Terminator5 : Terminator
  sen_GEO : Outport
  wires:
  Add2/1 -> sen_GEO/1
  Mux1/1 -> Add2/1
  Demux4/2 -> GEO_gain_tilt2/1
  Demux4/1 -> GEO_gain_tilt1/1
  Gain2/1 -> Mux1/2
  Ground/1 -> Mux1/3
  GEO_gain_tilt1/1 -> Mux1/1
  vel_GND/1 -> Demux4/1
  GEO_gain_tilt2/1 -> Gain2/1
  vel_F0/1 -> Demux1/1
  Demux1/1 -> GEO_gain/1
  Demux1/2 -> GEO_gain1/1
  Demux1/3 -> GEO_gain2/1
  GEO_gain/1 -> Mux2/1
  GEO_gain1/1 -> Mux2/2
  GEO_gain2/1 -> Mux2/3
  Mux2/1 -> Add2/2
  Demux4/3 -> Terminator5/1

== system ctrl_typeB/TypeB/SuspensionSystem/M_IFO_TM ==
  disp_TM : Inport
  Add2 : Sum  Inputs=++++
  Demux4 : Demux  Outputs=6
  Gain1 : Gain  Gain=1/300
  Gain2 : Gain  Gain=1e-3
  Gain3 : Gain  Gain=1e-3
  Terminator1 : Terminator
  Terminator3 : Terminator
  sen_IFO : Outport
  wires:
  disp_TM/1 -> Demux4/1
  Demux4/4 -> Terminator3/1
  Demux4/3 -> Gain1/1
  Demux4/2 -> Terminator1/1
  Add2/1 -> sen_IFO/1
  Demux4/1 -> Add2/1
  Gain1/1 -> Add2/2
  Demux4/5 -> Gain2/1
  Gain3/1 -> Add2/4
  Gain2/1 -> Add2/3
  Demux4/6 -> Gain3/1

== system ctrl_typeB/TypeB/SuspensionSystem/M_LVDT_F0 ==
  disp_GND : Inport
  disp_F0 : Inport  Port=2
  Add2 : Sum  Inputs=-+
  sen_LVDT : Outport
  wires:
  Add2/1 -> sen_LVDT/1
  disp_F0/1 -> Add2/2
  disp_GND/1 -> Add2/1

== system ctrl_typeB/TypeB/SuspensionSystem/M_LVDT_GAS ==
  disp_GAS : Inport
  Add1 : Sum  Inputs=-+
  Add2 : Sum  Inputs=-+
  Add3 : Sum  Inputs=-+
  Demux4 : Demux
  Mux3 : Mux  Inputs=3
  sen_LVDT : Outport
  wires:
  disp_GAS/1 -> Demux4/1
  Demux4/1 -> Add2/1
  Demux4/2 -> Add2/2, Add1/1
  Demux4/3 -> Add3/1, Add1/2
  Demux4/4 -> Add3/2
  Add2/1 -> Mux3/1
  Add1/1 -> Mux3/2
  Add3/1 -> Mux3/3
  Mux3/1 -> sen_LVDT/1

== system ctrl_typeB/TypeB/SuspensionSystem/M_OSEM_IM ==
  disp_IR : Inport
  disp_IM : Inport  Port=2
  Add1 : Sum
  Add2 : Sum  Inputs=+-
  Add3 : Sum  Inputs=-+
  Demux4 : Demux  Outputs=6
  Gain : Gain  Gain=76e-3
  Gain1 : Gain  Gain=76e-3
  Mux3 : Mux  Inputs=6
  sen_OSEM : Outport
  wires:
  disp_IM/1 -> Add3/2
  disp_IR/1 -> Demux4/1
  Demux4/6 -> Mux3/6
  Mux3/1 -> Add3/1
  Add3/1 -> sen_OSEM/1
  Demux4/1 -> Add2/1
  Demux4/2 -> Add1/1
  Demux4/3 -> Mux3/3
  Demux4/4 -> Gain/1, Mux3/4
  Demux4/5 -> Gain1/1, Mux3/5
  Gain1/1 -> Add2/2
  Gain/1 -> Add1/2
  Add1/1 -> Mux3/2
  Add2/1 -> Mux3/1

== system ctrl_typeB/TypeB/SuspensionSystem/M_OpLev_TM ==
  disp_TM : Inport
  Demux4 : Demux  Outputs=6
  Mux3 : Mux  Inputs=3
  Terminator1 : Terminator
  Terminator2 : Terminator
  Terminator3 : Terminator
  sen_OpLev : Outport
  wires:
  disp_TM/1 -> Demux4/1
  Mux3/1 -> sen_OpLev/1
  Demux4/4 -> Terminator3/1
  Demux4/3 -> Terminator2/1
  Demux4/2 -> Terminator1/1
  Demux4/1 -> Mux3/1
  Demux4/5 -> Mux3/2
  Demux4/6 -> Mux3/3

== system ctrl_typeB/TypeB/SuspensionSystem/M_act_GAS ==
  act_in : Inport
  Add1 : Sum  Inputs=+-
  Add2 : Sum  Inputs=+-
  Demux4 : Demux  Outputs=3
  Mux3 : Mux  Inputs=3
  act_out : Outport
  wires:
  act_in/1 -> Demux4/1
  Mux3/1 -> act_out/1
  Add1/1 -> Mux3/1
  Add2/1 -> Mux3/2
  Demux4/3 -> Mux3/3, Add2/2
  Demux4/2 -> Add1/2, Add2/1
  Demux4/1 -> Add1/1

== system ctrl_typeB/TypeB/SuspensionSystem/M_act_IM ==
  act_in : Inport
  Add1 : Sum  Inputs=-+
  Add2 : Sum
  Demux4 : Demux  Outputs=6
  Gain : Gain  Gain=76e-3
  Gain1 : Gain  Gain=76e-3
  Gain2 : Gain  Gain=-1
  Mux3 : Mux  Inputs=6
  act_out_IR : Outport
  act_out_IM : Outport  Port=2
  wires:
  act_in/1 -> Demux4/1, act_out_IM/1
  Gain1/1 -> Add2/1
  Gain/1 -> Add1/1
  Demux4/1 -> Mux3/1, Gain/1
  Demux4/2 -> Mux3/2, Gain1/1
  Demux4/4 -> Add2/2
  Demux4/5 -> Add1/2
  Demux4/3 -> Mux3/3
  Add2/1 -> Mux3/4
  Add1/1 -> Mux3/5
  Demux4/6 -> Mux3/6
  Mux3/1 -> Gain2/1
  Gain2/1 -> act_out_IR/1

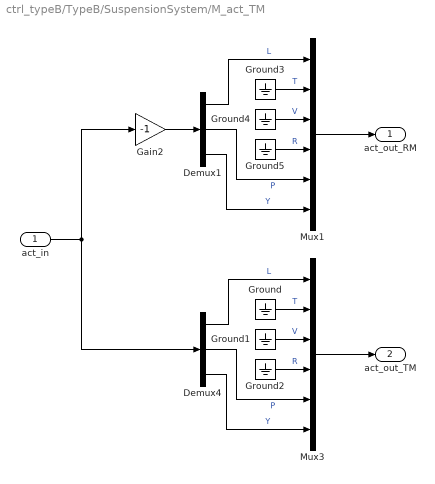
== system ctrl_typeB/TypeB/SuspensionSystem/M_act_TM ==
  act_in : Inport
  Demux1 : Demux  Outputs=3
  Demux4 : Demux  Outputs=3
  Gain2 : Gain  Gain=-1
  Ground{,1..5} (6 alike) : Ground
  Mux1 : Mux  Inputs=6
  Mux3 : Mux  Inputs=6
  act_out_RM : Outport
  act_out_TM : Outport  Port=2
  wires:
  act_in/1 -> Demux4/1, Gain2/1
  Gain2/1 -> Demux1/1
  Mux3/1 -> act_out_TM/1
  Demux4/1 -> Mux3/1  "L"
  Demux4/2 -> Mux3/5  "P"
  Demux4/3 -> Mux3/6  "Y"
  Ground/1 -> Mux3/2  "T"
  Ground1/1 -> Mux3/3  "V"
  Ground2/1 -> Mux3/4  "R"
  Mux1/1 -> act_out_RM/1
  Demux1/1 -> Mux1/1  "L"
  Demux1/2 -> Mux1/5  "P"
  Demux1/3 -> Mux1/6  "Y"
  Ground3/1 -> Mux1/2  "T"
  Ground4/1 -> Mux1/3  "V"
  Ground5/1 -> Mux1/4  "R"

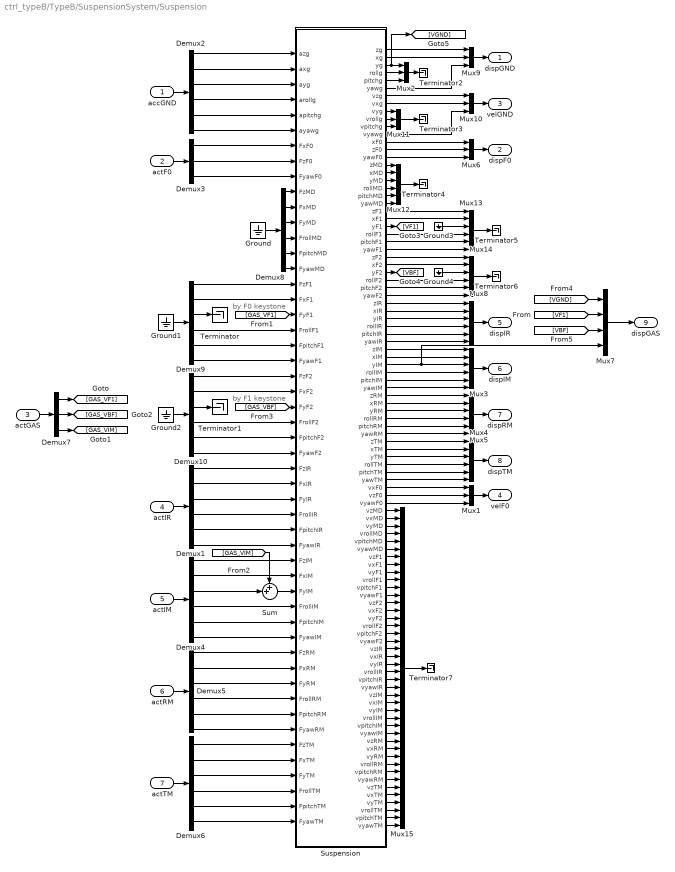
== system ctrl_typeB/TypeB/SuspensionSystem/Suspension ==
  note: by F0 keystone
  note: by F1 keystone
  accGND : Inport
  actF0 : Inport  Port=2
  actGAS : Inport  Port=3
  actIR : Inport  Port=4
  actIM : Inport  Port=5
  actRM : Inport  Port=6
  actTM : Inport  Port=7
  Demux{1..2,4..6,8..10} (8 alike) : Demux  Outputs=6
  Demux3 : Demux  Outputs=3
  Demux7 : Demux  Outputs=3
  Ground{,1..4} (5 alike) : Ground
  Mux{1..2,6,9..11} (6 alike) : Mux  Inputs=3
  Mux{3..5,8,12..14} (7 alike) : Mux  Inputs=6
  Mux15 : Mux  Inputs=42
  Mux7 : Mux
  Sum : Sum  Inputs=++|
  Suspension : Subsystem
  Terminator{,1..7} (8 alike) : Terminator
  dispGND : Outport
  dispF0 : Outport  Port=2
  velGND : Outport  Port=3
  velF0 : Outport  Port=4
  dispIR : Outport  Port=5
  dispIM : Outport  Port=6
  dispRM : Outport  Port=7
  dispTM : Outport  Port=8
  dispGAS : Outport  Port=9
  wires:
  actF0/1 -> Demux3/1
  accGND/1 -> Demux2/1
  actTM/1 -> Demux6/1
  actIR/1 -> Demux1/1
  actRM/1 -> Demux5/1
  actIM/1 -> Demux4/1
  Demux1/6 -> Suspension/33(FyawIR)
  Demux6/5 -> Suspension/50(FpitchTM)
  Demux1/5 -> Suspension/32(FpitchIR)
  Demux1/3 -> Suspension/30(FyIR)
  Demux1/1 -> Suspension/28(FzIR)
  Demux6/3 -> Suspension/48(FyTM)
  Demux4/2 -> Suspension/35(FxIM)
  Demux6/4 -> Suspension/49(FrollTM)
  Demux4/4 -> Suspension/37(FrollIM)
  Demux1/4 -> Suspension/31(FrollIR)
  Demux4/6 -> Suspension/39(FyawIM)
  Demux4/5 -> Suspension/38(FpitchIM)
  Demux4/1 -> Suspension/34(FzIM)
  Demux1/2 -> Suspension/29(FxIR)
  Demux6/1 -> Suspension/46(FzTM)
  Demux6/2 -> Suspension/47(FxTM)
  Demux6/6 -> Suspension/51(FyawTM)
  actGAS/1 -> Demux7/1
  Demux4/3 -> Sum/2
  Sum/1 -> Suspension/36(FyIM)
  Ground/1 -> Demux8/1
  Ground1/1 -> Demux9/1
  Demux7/3 -> [GAS_VIM]
  Demux7/1 -> [GAS_VF1]
  Demux7/2 -> [GAS_VBF]
  Demux2/1 -> Suspension/1(azg)
  Demux2/4 -> Suspension/4(arollg)
  Demux2/3 -> Suspension/3(ayg)
  Demux2/2 -> Suspension/2(axg)
  Demux2/6 -> Suspension/6(ayawg)
  Demux2/5 -> Suspension/5(apitchg)
  Demux3/1 -> Suspension/7(FxF0)
  Demux3/3 -> Suspension/9(FyawF0)
  Demux3/2 -> Suspension/8(FzF0)
  Demux8/1 -> Suspension/10(FzMD)
  Demux8/2 -> Suspension/11(FxMD)
  Demux8/4 -> Suspension/13(FrollMD)
  Demux8/6 -> Suspension/15(FyawMD)
  Demux8/3 -> Suspension/12(FyMD)
  Demux8/5 -> Suspension/14(FpitchMD)
  Demux9/1 -> Suspension/16(FzF1)
  Demux9/2 -> Suspension/17(FxF1)
  Demux9/4 -> Suspension/19(FrollF1)
  Demux9/6 -> Suspension/21(FyawF1)
  Demux9/5 -> Suspension/20(FpitchF1)
  [GAS_VF1] -> Suspension/18(FyF1)
  Demux9/3 -> Terminator/1
  Ground2/1 -> Demux10/1
  Demux10/1 -> Suspension/22(FzF2)
  Demux10/2 -> Suspension/23(FxF2)
  Demux10/4 -> Suspension/25(FrollF2)
  Demux10/6 -> Suspension/27(FyawF2)
  Demux10/5 -> Suspension/26(FpitchF2)
  Demux10/3 -> Terminator1/1
  [GAS_VBF] -> Suspension/24(FyF2)
  Demux5/1 -> Suspension/40(FzRM)
  Demux5/2 -> Suspension/41(FxRM)
  Demux5/3 -> Suspension/42(FyRM)
  Demux5/4 -> Suspension/43(FrollRM)
  Demux5/5 -> Suspension/44(FpitchRM)
  Demux5/6 -> Suspension/45(FyawRM)
  Mux9/1 -> dispGND/1
  Suspension/1(zg) -> Mux9/1
  Suspension/2(xg) -> Mux9/2
  Suspension/6(yawg) -> Mux9/3
  Suspension/3(yg) -> [VGND], Mux2/1
  Suspension/4(rollg) -> Mux2/2
  Suspension/5(pitchg) -> Mux2/3
  Mux10/1 -> velGND/1
  Suspension/7(vzg) -> Mux10/1
  Suspension/8(vxg) -> Mux10/2
  Suspension/12(vyawg) -> Mux10/3
  Suspension/9(vyg) -> Mux11/1
  Suspension/10(vrollg) -> Mux11/2
  Suspension/11(vpitchg) -> Mux11/3
  Mux6/1 -> dispF0/1
  Suspension/13(xF0) -> Mux6/1
  Suspension/14(zF0) -> Mux6/2
  Suspension/15(yawF0) -> Mux6/3
  Suspension/16(zMD) -> Mux12/1
  Suspension/17(xMD) -> Mux12/2
  Suspension/18(yMD) -> Mux12/3
  Suspension/19(rollMD) -> Mux12/4
  Suspension/21(yawMD) -> Mux12/6
  Suspension/20(pitchMD) -> Mux12/5
  Mux3/1 -> dispIM/1
  Mux8/1 -> dispIR/1
  Mux4/1 -> dispTM/1
  Mux5/1 -> dispRM/1
  Suspension/57(yawTM) -> Mux4/6
  Suspension/52(zTM) -> Mux4/1
  Suspension/53(xTM) -> Mux4/2
  Suspension/54(yTM) -> Mux4/3
  Suspension/55(rollTM) -> Mux4/4
  Suspension/56(pitchTM) -> Mux4/5
  Suspension/40(zIM) -> Mux3/1
  Suspension/41(xIM) -> Mux3/2
  Suspension/42(yIM) -> Mux3/3, Mux7/4
  Suspension/43(rollIM) -> Mux3/4
  Suspension/44(pitchIM) -> Mux3/5
  Suspension/45(yawIM) -> Mux3/6
  Suspension/34(zIR) -> Mux8/1
  Suspension/35(xIR) -> Mux8/2
  Suspension/36(yIR) -> Mux8/3
  Suspension/37(rollIR) -> Mux8/4
  Suspension/38(pitchIR) -> Mux8/5
  Suspension/39(yawIR) -> Mux8/6
  Suspension/24(yF1) -> [VF1]
  Mux7/1 -> dispGAS/1
  Suspension/46(zRM) -> Mux5/1
  Suspension/47(xRM) -> Mux5/2
  Suspension/48(yRM) -> Mux5/3
  Suspension/49(rollRM) -> Mux5/4
  Suspension/50(pitchRM) -> Mux5/5
  Suspension/51(yawRM) -> Mux5/6
  Mux1/1 -> velF0/1
  Suspension/58(vxF0) -> Mux1/1
  Suspension/59(vzF0) -> Mux1/2
  Suspension/60(vyawF0) -> Mux1/3
  Mux2/1 -> Terminator2/1
  Mux11/1 -> Terminator3/1
  Mux12/1 -> Terminator4/1
  Mux13/1 -> Terminator5/1
  Suspension/23(xF1) -> Mux13/2
  Suspension/25(rollF1) -> Mux13/4
  Suspension/26(pitchF1) -> Mux13/5
  Suspension/27(yawF1) -> Mux13/6
  Suspension/22(zF1) -> Mux13/1
  Ground3/1 -> Mux13/3
  Mux14/1 -> Terminator6/1
  Suspension/29(xF2) -> Mux14/2
  Suspension/31(rollF2) -> Mux14/4
  Suspension/32(pitchF2) -> Mux14/5
  Suspension/33(yawF2) -> Mux14/6
  Suspension/28(zF2) -> Mux14/1
  Ground4/1 -> Mux14/3
  Suspension/30(yF2) -> [VBF]
  [VGND] -> Mux7/1
  [VF1] -> Mux7/2
  [VBF] -> Mux7/3
  Suspension/76(vrollF2) -> Mux15/16
  Suspension/77(vpitchF2) -> Mux15/17
  Suspension/92(vxRM) -> Mux15/32
  Suspension/93(vyRM) -> Mux15/33
  Suspension/96(vyawRM) -> Mux15/36
  Suspension/97(vzTM) -> Mux15/37
  Suspension/94(vrollRM) -> Mux15/34
  Suspension/95(vpitchRM) -> Mux15/35
  Suspension/82(vrollIR) -> Mux15/22
  Suspension/83(vpitchIR) -> Mux15/23
  Suspension/86(vxIM) -> Mux15/26
  Suspension/87(vyIM) -> Mux15/27
  Suspension/84(vyawIR) -> Mux15/24
  Suspension/85(vzIM) -> Mux15/25
  Suspension/88(vrollIM) -> Mux15/28
  Suspension/89(vpitchIM) -> Mux15/29
  Suspension/90(vyawIM) -> Mux15/30
  Suspension/91(vzRM) -> Mux15/31
  Suspension/72(vyawF1) -> Mux15/12
  Suspension/73(vzF2) -> Mux15/13
  Suspension/74(vxF2) -> Mux15/14
  Suspension/75(vyF2) -> Mux15/15
  Suspension/68(vxF1) -> Mux15/8
  Suspension/69(vyF1) -> Mux15/9
  Suspension/70(vrollF1) -> Mux15/10
  Suspension/71(vpitchF1) -> Mux15/11
  Suspension/80(vxIR) -> Mux15/20
  Suspension/81(vyIR) -> Mux15/21
  Suspension/78(vyawF2) -> Mux15/18
  Suspension/79(vzIR) -> Mux15/19
  Suspension/100(vrollTM) -> Mux15/40
  Suspension/101(vpitchTM) -> Mux15/41
  Suspension/102(vyawTM) -> Mux15/42
  Suspension/98(vxTM) -> Mux15/38
  Suspension/99(vyTM) -> Mux15/39
  Suspension/64(vrollMD) -> Mux15/4
  Suspension/65(vpitchMD) -> Mux15/5
  Suspension/62(vxMD) -> Mux15/2
  Suspension/63(vyMD) -> Mux15/3
  Suspension/66(vyawMD) -> Mux15/6
  Suspension/67(vzF1) -> Mux15/7
  Suspension/61(vzMD) -> Mux15/1
  Mux15/1 -> Terminator7/1
  [GAS_VIM] -> Sum/1

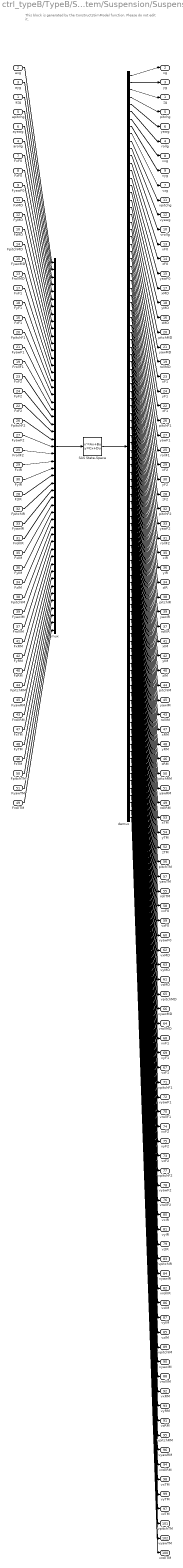
== system ctrl_typeB/TypeB/SuspensionSystem/Suspension/Suspension ==
  note: This block is generated by the ConstructsSimModel function.
      | Please do not edit it.
  azg : Inport
  axg : Inport  Port=2
  ayg : Inport  Port=3
  arollg : Inport  Port=4
  apitchg : Inport  Port=5
  ayawg : Inport  Port=6
  FxF0 : Inport  Port=7
  FzF0 : Inport  Port=8
  FyawF0 : Inport  Port=9
  FzMD : Inport  Port=10
  FxMD : Inport  Port=11
  FyMD : Inport  Port=12
  FrollMD : Inport  Port=13
  FpitchMD : Inport  Port=14
  FyawMD : Inport  Port=15
  FzF1 : Inport  Port=16
  FxF1 : Inport  Port=17
  FyF1 : Inport  Port=18
  FrollF1 : Inport  Port=19
  FpitchF1 : Inport  Port=20
  FyawF1 : Inport  Port=21
  FzF2 : Inport  Port=22
  FxF2 : Inport  Port=23
  FyF2 : Inport  Port=24
  FrollF2 : Inport  Port=25
  FpitchF2 : Inport  Port=26
  FyawF2 : Inport  Port=27
  FzIR : Inport  Port=28
  FxIR : Inport  Port=29
  FyIR : Inport  Port=30
  FrollIR : Inport  Port=31
  FpitchIR : Inport  Port=32
  FyawIR : Inport  Port=33
  FzIM : Inport  Port=34
  FxIM : Inport  Port=35
  FyIM : Inport  Port=36
  FrollIM : Inport  Port=37
  FpitchIM : Inport  Port=38
  FyawIM : Inport  Port=39
  FzRM : Inport  Port=40
  FxRM : Inport  Port=41
  FyRM : Inport  Port=42
  FrollRM : Inport  Port=43
  FpitchRM : Inport  Port=44
  FyawRM : Inport  Port=45
  FzTM : Inport  Port=46
  FxTM : Inport  Port=47
  FyTM : Inport  Port=48
  FrollTM : Inport  Port=49
  FpitchTM : Inport  Port=50
  FyawTM : Inport  Port=51
  SAS State-Space : StateSpace  A=sys1.A  B=sys1.B  C=sys1.C  D=sys1.D  X0=0  ContinuousStateAttributes='SUS_SS_MODEL'
  demux : Demux  Outputs=102
  mux : Mux  Inputs=51
  zg : Outport
  xg : Outport  Port=2
  yg : Outport  Port=3
  rollg : Outport  Port=4
  pitchg : Outport  Port=5
  yawg : Outport  Port=6
  vzg : Outport  Port=7
  vxg : Outport  Port=8
  vyg : Outport  Port=9
  vrollg : Outport  Port=10
  vpitchg : Outport  Port=11
  vyawg : Outport  Port=12
  xF0 : Outport  Port=13
  zF0 : Outport  Port=14
  yawF0 : Outport  Port=15
  zMD : Outport  Port=16
  xMD : Outport  Port=17
  yMD : Outport  Port=18
  rollMD : Outport  Port=19
  pitchMD : Outport  Port=20
  yawMD : Outport  Port=21
  zF1 : Outport  Port=22
  xF1 : Outport  Port=23
  yF1 : Outport  Port=24
  rollF1 : Outport  Port=25
  pitchF1 : Outport  Port=26
  yawF1 : Outport  Port=27
  zF2 : Outport  Port=28
  xF2 : Outport  Port=29
  yF2 : Outport  Port=30
  rollF2 : Outport  Port=31
  pitchF2 : Outport  Port=32
  yawF2 : Outport  Port=33
  zIR : Outport  Port=34
  xIR : Outport  Port=35
  yIR : Outport  Port=36
  rollIR : Outport  Port=37
  pitchIR : Outport  Port=38
  yawIR : Outport  Port=39
  zIM : Outport  Port=40
  xIM : Outport  Port=41
  yIM : Outport  Port=42
  rollIM : Outport  Port=43
  pitchIM : Outport  Port=44
  yawIM : Outport  Port=45
  zRM : Outport  Port=46
  xRM : Outport  Port=47
  yRM : Outport  Port=48
  rollRM : Outport  Port=49
  pitchRM : Outport  Port=50
  yawRM : Outport  Port=51
  zTM : Outport  Port=52
  xTM : Outport  Port=53
  yTM : Outport  Port=54
  rollTM : Outport  Port=55
  pitchTM : Outport  Port=56
  yawTM : Outport  Port=57
  vxF0 : Outport  Port=58
  vzF0 : Outport  Port=59
  vyawF0 : Outport  Port=60
  vzMD : Outport  Port=61
  vxMD : Outport  Port=62
  vyMD : Outport  Port=63
  vrollMD : Outport  Port=64
  vpitchMD : Outport  Port=65
  vyawMD : Outport  Port=66
  vzF1 : Outport  Port=67
  vxF1 : Outport  Port=68
  vyF1 : Outport  Port=69
  vrollF1 : Outport  Port=70
  vpitchF1 : Outport  Port=71
  vyawF1 : Outport  Port=72
  vzF2 : Outport  Port=73
  vxF2 : Outport  Port=74
  vyF2 : Outport  Port=75
  vrollF2 : Outport  Port=76
  vpitchF2 : Outport  Port=77
  vyawF2 : Outport  Port=78
  vzIR : Outport  Port=79
  vxIR : Outport  Port=80
  vyIR : Outport  Port=81
  vrollIR : Outport  Port=82
  vpitchIR : Outport  Port=83
  vyawIR : Outport  Port=84
  vzIM : Outport  Port=85
  vxIM : Outport  Port=86
  vyIM : Outport  Port=87
  vrollIM : Outport  Port=88
  vpitchIM : Outport  Port=89
  vyawIM : Outport  Port=90
  vzRM : Outport  Port=91
  vxRM : Outport  Port=92
  vyRM : Outport  Port=93
  vrollRM : Outport  Port=94
  vpitchRM : Outport  Port=95
  vyawRM : Outport  Port=96
  vzTM : Outport  Port=97
  vxTM : Outport  Port=98
  vyTM : Outport  Port=99
  vrollTM : Outport  Port=100
  vpitchTM : Outport  Port=101
  vyawTM : Outport  Port=102
  wires:
  mux/1 -> SAS State-Space/1
  SAS State-Space/1 -> demux/1
  axg/1 -> mux/1
  ayg/1 -> mux/2
  azg/1 -> mux/3
  apitchg/1 -> mux/4
  ayawg/1 -> mux/5
  arollg/1 -> mux/6
  FxF0/1 -> mux/7
  FzF0/1 -> mux/8
  FyawF0/1 -> mux/9
  FxMD/1 -> mux/10
  FyMD/1 -> mux/11
  FzMD/1 -> mux/12
  FpitchMD/1 -> mux/13
  FyawMD/1 -> mux/14
  FrollMD/1 -> mux/15
  FxF1/1 -> mux/16
  FyF1/1 -> mux/17
  FzF1/1 -> mux/18
  FpitchF1/1 -> mux/19
  FyawF1/1 -> mux/20
  FrollF1/1 -> mux/21
  FxF2/1 -> mux/22
  FyF2/1 -> mux/23
  FzF2/1 -> mux/24
  FpitchF2/1 -> mux/25
  FyawF2/1 -> mux/26
  FrollF2/1 -> mux/27
  FxIR/1 -> mux/28
  FyIR/1 -> mux/29
  FzIR/1 -> mux/30
  FpitchIR/1 -> mux/31
  FyawIR/1 -> mux/32
  FrollIR/1 -> mux/33
  FxIM/1 -> mux/34
  FyIM/1 -> mux/35
  FzIM/1 -> mux/36
  FpitchIM/1 -> mux/37
  FyawIM/1 -> mux/38
  FrollIM/1 -> mux/39
  FxRM/1 -> mux/40
  FyRM/1 -> mux/41
  FzRM/1 -> mux/42
  FpitchRM/1 -> mux/43
  FyawRM/1 -> mux/44
  FrollRM/1 -> mux/45
  FxTM/1 -> mux/46
  FyTM/1 -> mux/47
  FzTM/1 -> mux/48
  FpitchTM/1 -> mux/49
  FyawTM/1 -> mux/50
  FrollTM/1 -> mux/51
  demux/1 -> xg/1
  demux/2 -> yg/1
  demux/3 -> zg/1
  demux/4 -> pitchg/1
  demux/5 -> yawg/1
  demux/6 -> rollg/1
  demux/7 -> vxg/1
  demux/8 -> vyg/1
  demux/9 -> vzg/1
  demux/10 -> vpitchg/1
  demux/11 -> vyawg/1
  demux/12 -> vrollg/1
  demux/13 -> xF0/1
  demux/14 -> zF0/1
  demux/15 -> yawF0/1
  demux/16 -> xMD/1
  demux/17 -> yMD/1
  demux/18 -> zMD/1
  demux/19 -> pitchMD/1
  demux/20 -> yawMD/1
  demux/21 -> rollMD/1
  demux/22 -> xF1/1
  demux/23 -> yF1/1
  demux/24 -> zF1/1
  demux/25 -> pitchF1/1
  demux/26 -> yawF1/1
  demux/27 -> rollF1/1
  demux/28 -> xF2/1
  demux/29 -> yF2/1
  demux/30 -> zF2/1
  demux/31 -> pitchF2/1
  demux/32 -> yawF2/1
  demux/33 -> rollF2/1
  demux/34 -> xIR/1
  demux/35 -> yIR/1
  demux/36 -> zIR/1
  demux/37 -> pitchIR/1
  demux/38 -> yawIR/1
  demux/39 -> rollIR/1
  demux/40 -> xIM/1
  demux/41 -> yIM/1
  demux/42 -> zIM/1
  demux/43 -> pitchIM/1
  demux/44 -> yawIM/1
  demux/45 -> rollIM/1
  demux/46 -> xRM/1
  demux/47 -> yRM/1
  demux/48 -> zRM/1
  demux/49 -> pitchRM/1
  demux/50 -> yawRM/1
  demux/51 -> rollRM/1
  demux/52 -> xTM/1
  demux/53 -> yTM/1
  demux/54 -> zTM/1
  demux/55 -> pitchTM/1
  demux/56 -> yawTM/1
  demux/57 -> rollTM/1
  demux/58 -> vxF0/1
  demux/59 -> vzF0/1
  demux/60 -> vyawF0/1
  demux/61 -> vxMD/1
  demux/62 -> vyMD/1
  demux/63 -> vzMD/1
  demux/64 -> vpitchMD/1
  demux/65 -> vyawMD/1
  demux/66 -> vrollMD/1
  demux/67 -> vxF1/1
  demux/68 -> vyF1/1
  demux/69 -> vzF1/1
  demux/70 -> vpitchF1/1
  demux/71 -> vyawF1/1
  demux/72 -> vrollF1/1
  demux/73 -> vxF2/1
  demux/74 -> vyF2/1
  demux/75 -> vzF2/1
  demux/76 -> vpitchF2/1
  demux/77 -> vyawF2/1
  demux/78 -> vrollF2/1
  demux/79 -> vxIR/1
  demux/80 -> vyIR/1
  demux/81 -> vzIR/1
  demux/82 -> vpitchIR/1
  demux/83 -> vyawIR/1
  demux/84 -> vrollIR/1
  demux/85 -> vxIM/1
  demux/86 -> vyIM/1
  demux/87 -> vzIM/1
  demux/88 -> vpitchIM/1
  demux/89 -> vyawIM/1
  demux/90 -> vrollIM/1
  demux/91 -> vxRM/1
  demux/92 -> vyRM/1
  demux/93 -> vzRM/1
  demux/94 -> vpitchRM/1
  demux/95 -> vyawRM/1
  demux/96 -> vrollRM/1
  demux/97 -> vxTM/1
  demux/98 -> vyTM/1
  demux/99 -> vzTM/1
  demux/100 -> vpitchTM/1
  demux/101 -> vyawTM/1
  demux/102 -> vrollTM/1
